simulink model "Exp6_simulink"  (R2015a)
settings: Solver=ode45  StartTime=0.0  StopTime=10  RelTol=1e-3
values from neighbouring files (symbols this model uses):
  degrau = wm/K    (= 1.7129699802)    [exp6.m]
  K = 55.0201    [exp6.m]
  KNL = 59.85    [exp6.m]
  Kp = 1.455    [exp6.m]
  Kpi = 4    [exp6.m]
  Kt = 0.0169    [exp6.m]
  phi = 1.2    [exp6.m]
  T = 0.27    [exp6.m]
  Ti = T    (= 0.27)    [exp6.m]
settings Model: Creator=anton  LastModifiedBy=duane

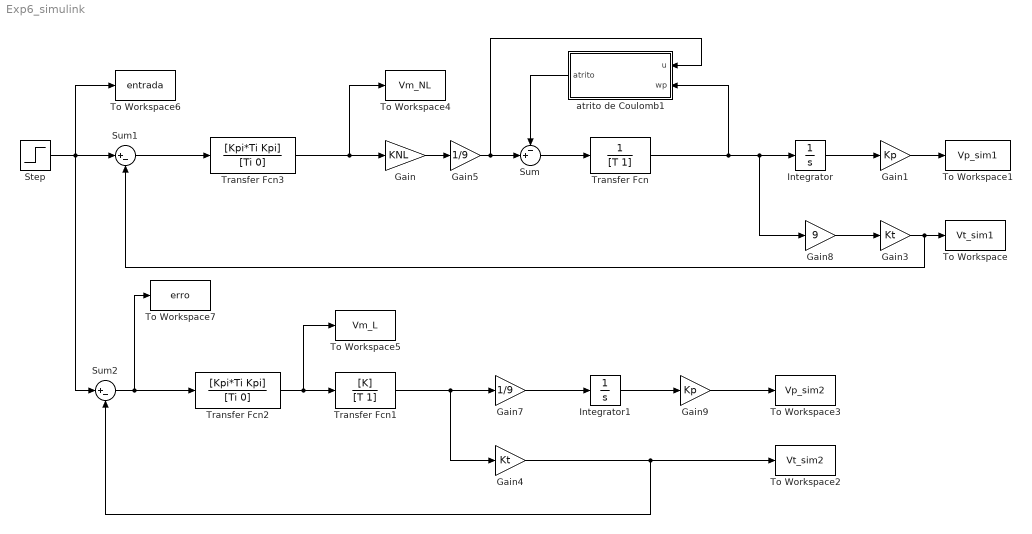
== system Exp6_simulink ==
  Gain : Gain  Gain=KNL
  Gain1 : Gain  Gain=Kp
  Gain3 : Gain  Gain=Kt
  Gain4 : Gain  Gain=Kt
  Gain5 : Gain  Gain=1/9
  Gain7 : Gain  Gain=1/9
  Gain8 : Gain  Gain=9
  Gain9 : Gain  Gain=Kp
  Integrator : Integrator
  Integrator1 : Integrator
  Step : Step  After=degrau  SampleTime=0.01
  Sum : Sum  Inputs=-+|
  Sum1 : Sum  Inputs=|+-
  Sum2 : Sum  Inputs=|+-
  To Workspace : ToWorkspace  VariableName=Vt_sim1  SampleTime=-1
  To Workspace1 : ToWorkspace  VariableName=Vp_sim1  SampleTime=-1
  To Workspace2 : ToWorkspace  VariableName=Vt_sim2  SampleTime=-1
  To Workspace3 : ToWorkspace  VariableName=Vp_sim2  SampleTime=-1
  To Workspace4 : ToWorkspace  VariableName=Vm_NL  SampleTime=-1
  To Workspace5 : ToWorkspace  VariableName=Vm_L  SampleTime=-1
  To Workspace6 : ToWorkspace  VariableName=entrada  SampleTime=-1
  To Workspace7 : ToWorkspace  VariableName=erro  SampleTime=-1
  Transfer Fcn : TransferFcn  Denominator=[T 1]
  Transfer Fcn1 : TransferFcn  Numerator=[K]  Denominator=[T 1]
  Transfer Fcn2 : TransferFcn  Numerator=[Kpi*Ti Kpi]  Denominator=[Ti 0]
  Transfer Fcn3 : TransferFcn  Numerator=[Kpi*Ti Kpi]  Denominator=[Ti 0]
  atrito de Coulomb1 : Subsystem  mask{phi=phi}
      mask Display: fprintf('phi = %3.1f', phi)
  wires:
  Gain/1 -> Gain5/1
  Transfer Fcn/1 -> atrito de Coulomb1/2(wp), Gain8/1, Integrator/1
  Integrator/1 -> Gain1/1
  Sum1/1 -> Transfer Fcn3/1
  Transfer Fcn3/1 -> To Workspace4/1, Gain/1
  Gain3/1 -> To Workspace/1, Sum1/2
  Gain1/1 -> To Workspace1/1
  Gain8/1 -> Gain3/1
  Sum/1 -> Transfer Fcn/1
  Gain5/1 -> atrito de Coulomb1/1(u), Sum/2
  Transfer Fcn1/1 -> Gain4/1, Gain7/1
  Gain7/1 -> Integrator1/1
  Integrator1/1 -> Gain9/1
  Gain9/1 -> To Workspace3/1
  Gain4/1 -> To Workspace2/1, Sum2/2
  Sum2/1 -> Transfer Fcn2/1, To Workspace7/1
  Transfer Fcn2/1 -> To Workspace5/1, Transfer Fcn1/1
  Step/1 -> To Workspace6/1, Sum2/1, Sum1/1
  atrito de Coulomb1/1(atrito) -> Sum/1

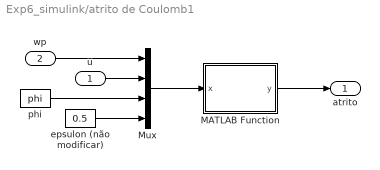
== system Exp6_simulink/atrito de Coulomb1 ==
  u : Inport
  wp : Inport  Port=2
  MATLAB Function : MATLAB Function  TreatAsAtomicUnit=on
  Mux : Mux
  epsulon (não modificar) : Constant  Value=0.5
  phi : Constant  Value=phi
  atrito : Outport
  wires:
  u/1 -> Mux/2
  phi/1 -> Mux/3
  MATLAB Function/1(y) -> atrito/1
  wp/1 -> Mux/1
  epsulon (não modificar)/1 -> Mux/4
  Mux/1 -> MATLAB Function/1(x)

== matlab function Exp6_simulink/atrito de Coulomb1/MATLAB Function ==
  data: x input size=4; y output size=1
function y = nl_coulomb(x)
% Atrito de Coulomb
% Para uso de nl_template.mdl

wp  = x(1); 
u   = x(2); 
phi = x(3); 
epsulon = x(4);

y = 0;

if wp > epsulon
    y = phi;
elseif wp < -epsulon
    y = -phi;
elseif wp >= 0
    y = min(phi,abs(u));
elseif wp < 0
    y = max(-phi,-abs(u));
end
